simulink model "sampleModel366"  (R2021b)
settings: Solver=VariableStepAuto  StartTime=0.0  StopTime=10.0  RelTol=1e-3
undefined symbols (not defined in the file or in its folder): magnitude, Newton, Raphson
libraries: simulink x7, slpidlib x1
settings Model: Creator=user  LastModifiedBy=user

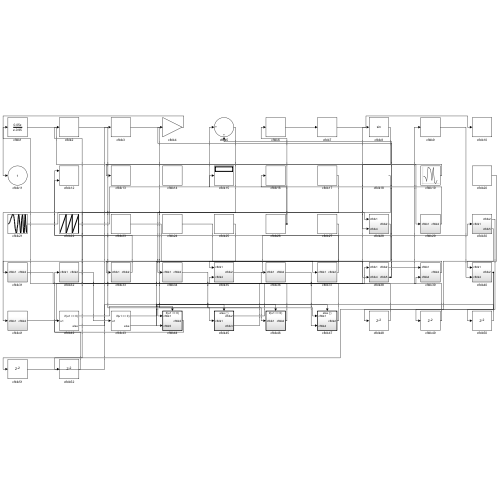
[thumbnail: Simulink's stored preview of the top-level diagram]
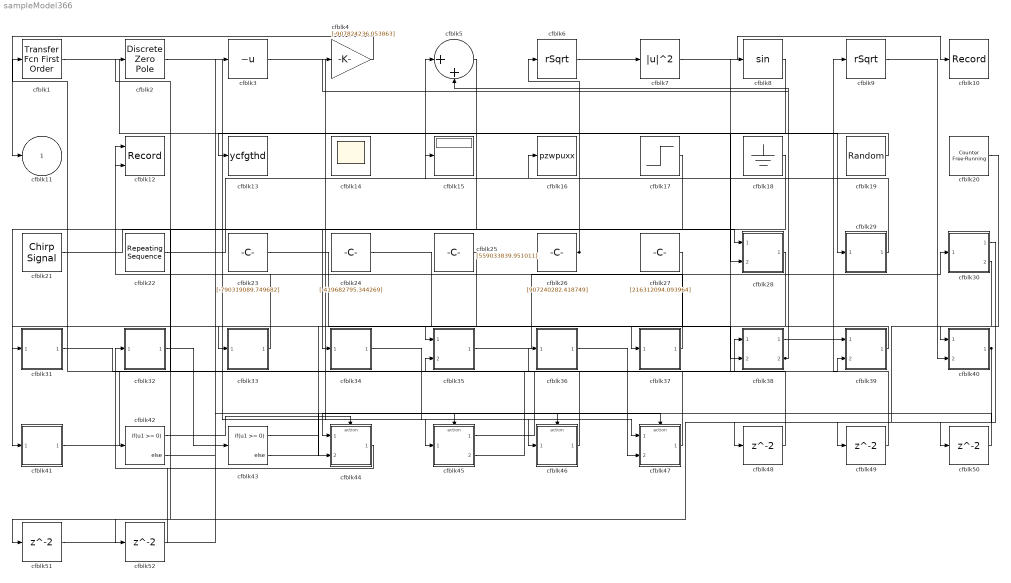
== system sampleModel366 ==
  cfblk1 : simulink/Discrete/Transfer Fcn First Order  PoleZ=0.95  ICPrevOutput=0.0  DoSatur=off
  cfblk10 : Record  FileSettingsInternal="{\"entries\":[{\"content\":{\"excelSettings\":{\"content\":{},\"type\":\"Streamout.ExcelSettings\"}},\"type\":\"Streamout.FileSettingStorage\",\"uuid\":\"b8f6fc41-c9ad-439a-b2d6-c8baa77482f0\"}],\"packageUris\":[\"http://schema.mathworks.com/mf0/streamout_blocks/R2020a\"],\"version\":\"1.0\"}"  SignalsInternal="{\"entries\":[{\"content\":{\"signals\":[{\"content\":{\"blockPath\":[\"sampleModel366/cfblk10\"],\"channel\":[],\"dimensions\":[1],\"domain\":\"sampleModel366/cfblk10\",\"lineColor\":\"#77ac30\",\"plots\":[1],\"port\":1,\"sid\":[\"\"],\"signalID\":15171,\"signalName\":\"cfblk7\"},\"type\":\"RecordBlkView.Signal\",\"uuid\":\"9359990c-ce8d-4281-8ced-0906e446bae2\"}]},\"type\":\"RecordBlkView.InputSignals\",\"uuid\":\"4aa2d466-194c-4383-9850-03db0f9c61d1\"}],\"packageUris\":[\"http://schema.mathworks.com/mf0/streamout_blocks/R2020a\"],\"version\":\"1.0\"}"  VisualizationBindings="{\"sparklinesplugin\":{\"info\":[{\"bindingParametersList\":[],\"subplotID\":1}]}}"
  cfblk12 : Record  FileSettingsInternal="{\"entries\":[{\"content\":{\"excelSettings\":{\"content\":{},\"type\":\"Streamout.ExcelSettings\"}},\"type\":\"Streamout.FileSettingStorage\",\"uuid\":\"68a24281-bd12-4afd-970e-6bf11612f610\"}],\"packageUris\":[\"http://schema.mathworks.com/mf0/streamout_blocks/R2020a\"],\"version\":\"1.0\"}"  Layout=[1 1]  SignalsInternal="{\"entries\":[{\"content\":{\"signals\":[{\"content\":{\"blockPath\":[\"sampleModel366/cfblk12\"],\"channel\":[],\"dimensions\":[1],\"domain\":\"sampleModel366/cfblk12\",\"lineColor\":\"#a2142f\",\"plots\":[1],\"port\":1,\"sid\":[\"\"],\"signalID\":15175,\"signalName\":\"cfblk37\"},\"type\":\"RecordBlkView.Signal\",\"uuid\":\"ee091272-d34b-41c7-8e6f-0fe17ae82c56\"},{\"content\":{\"blockPath\":[\"sampleModel366/cfblk12\"],\"channel\":[],\"dimensions\":[1],\"domain\":\"sampleModel366/cfblk12\",\"lineColor\":\"#139fff\",\"plots\":[1],\"port\":2,\"sid\":[\"\"],\"signalID\":15179,\"signalName\":\"cfblk33\"},\"type\":\"RecordBlkView.Signal\",\"uuid\":\"8b8a614a-960d-4b88-85a9-f6698a1653c2\"}]},\"type\":\"RecordBlkView.InputSignals\",\"uuid\":\"fcbbfd92-8274-4e20-9f39-c881c6846dea\"}],\"packageUris\":[\"http://schema.mathworks.com/mf0/streamout_blocks/R2020a\"],\"version\":\"1.0\"}"  VisualizationBindings="{\"xyplotplugin\":{\"info\":[{\"series\":[{\"bindingParametersList\":[{\"parameter\":\"X-Axis\",\"signalID\":15175,\"signalName\":\"cfblk37\"},{\"parameter\":\"Y-Axis\",\"signalID\":15179,\"signalName\":\"cfblk33\"}],\"seriesID\":23164}],\"subplotID\":1}]}}"  CompatibilityTag=XY
  cfblk13 : ToWorkspace  VariableName=ycfgthd  SaveFormat=Timeseries  SampleTime=-1
  cfblk14 : Scope
      settings: Floating=on
  cfblk15 : Display
  cfblk16 : ToWorkspace  VariableName=pzwpuxx  SaveFormat=Timeseries  SampleTime=-1
  cfblk17 : Step  Time=[5.000000]  Before=[178683344.473768]  After=[-623757983.996930]  SampleTime=0
  cfblk18 : Ground
  cfblk19 : RandomNumber  Mean=[-66694.921221]  Variance=[14545.838381]  Seed=[878185386.000000]  SampleTime=0.1
  cfblk2 : DiscreteZeroPole  Poles=[0 0.5]  Gain=1
  cfblk20 : simulink/Sources/Counter Free-Running  NumBits=[58.000000]  tsamp=-1
  cfblk21 : simulink/Sources/Chirp Signal  f1=[528864126.844984]  T=[-218465331.060448]  f2=[-783705554.218614]
  cfblk22 : simulink/Sources/Repeating Sequence  rep_seq_t=[0 2]  rep_seq_y=[169942996.806299, 363068189.269471]
  cfblk23 : Constant  Value=[-790319089.749682]  SampleTime=1
  cfblk24 : Constant  Value=[-419682795.344269]  SampleTime=1
  cfblk25 : Constant  Value=[559033839.951011]  SampleTime=1
  cfblk26 : Constant  Value=[907240282.418749]  SampleTime=1
  cfblk27 : Constant  Value=[216312094.093964]  SampleTime=1
  cfblk28 : Subsystem
  cfblk29 : Subsystem
  cfblk3 : UnaryMinus
  cfblk30 : Subsystem
  cfblk31 : Subsystem
  cfblk32 : Subsystem
  cfblk33 : Subsystem
  cfblk34 : Subsystem
  cfblk35 : Subsystem
  cfblk36 : Subsystem
  cfblk37 : Subsystem
  cfblk38 : Subsystem
  cfblk39 : Subsystem
  cfblk4 : Gain  Gain=[-907824236.053863]
  cfblk40 : Subsystem
  cfblk41 : Subsystem
  cfblk42 : If  IfExpression=u1 >= 0  SampleTime=1
  cfblk43 : If  IfExpression=u1 >= 0  SampleTime=1
  cfblk44 : Subsystem  TreatAsAtomicUnit=on
  cfblk45 : Subsystem  TreatAsAtomicUnit=on
  cfblk46 : Subsystem  TreatAsAtomicUnit=on
  cfblk47 : Subsystem  TreatAsAtomicUnit=on
  cfblk{48..52} (5 alike) : Delay  SampleTime=1
  cfblk5 : Sum  Inputs=|++
  cfblk6 : Sqrt  Operator=rSqrt  AlgorithmType=Newton-Raphson  SaturateOnIntegerOverflow=on
  cfblk7 : Math  Operator=magnitude^2  SaturateOnIntegerOverflow=on
  cfblk8 : Trigonometry
  cfblk9 : Sqrt  Operator=rSqrt  AlgorithmType=Newton-Raphson  SaturateOnIntegerOverflow=on
  cfblk11 : Outport
  wires:
  cfblk39/1(cfblk2) -> cfblk35/1(cfblk1)
  cfblk29/1(cfblk2) -> cfblk16/1
  cfblk2/1 -> cfblk47/1(cfblk1)
  cfblk7/1 -> cfblk10/1
  cfblk19/1 -> cfblk13/1
  cfblk44/1(cfblk2) -> cfblk32/1(cfblk1)
  cfblk6/1 -> cfblk7/1
  cfblk3/1 -> cfblk45/1(cfblk1)
  cfblk17/1 -> cfblk34/1(cfblk1)
  cfblk21/1 -> cfblk28/1(cfblk1)
  cfblk32/1(cfblk2) -> cfblk43/1
  cfblk22/1 -> cfblk5/1
  cfblk8/1 -> cfblk28/2(cfblk4)
  cfblk37/1(cfblk2) -> cfblk12/1
  cfblk1/1 -> cfblk29/1(cfblk1)
  cfblk36/1(cfblk2) -> cfblk47/2(cfblk4)
  cfblk4/1 -> cfblk11/1
  cfblk40/1(cfblk2) -> cfblk50/1, cfblk51/1
  cfblk24/1 -> cfblk37/1(cfblk1)
  cfblk18/1 -> cfblk41/1(cfblk1)
  cfblk46/1(cfblk2) -> cfblk2/1
  cfblk25/1 -> cfblk33/1(cfblk1)
  cfblk38/1(cfblk2) -> cfblk9/1
  cfblk27/1 -> cfblk44/2(cfblk5)
  cfblk20/1 -> cfblk40/1(cfblk1)
  cfblk26/1 -> cfblk15/1, cfblk6/1
  cfblk28/1(cfblk2) -> cfblk31/1(cfblk1)
  cfblk35/1(cfblk2) -> cfblk30/1(cfblk1)
  cfblk38/2(cfblk5) -> cfblk5/2, cfblk4/1
  cfblk47/1(cfblk2) -> cfblk1/1
  cfblk9/1 -> cfblk40/2(cfblk4)
  cfblk45/1(cfblk2) -> cfblk8/1
  cfblk33/1(cfblk2) -> cfblk12/2
  cfblk34/1(cfblk2) -> cfblk46/1(cfblk1)
  cfblk41/1(cfblk2) -> cfblk36/1(cfblk1)
  cfblk45/2(cfblk3) -> cfblk38/1(cfblk1)
  cfblk23/1 -> cfblk38/2(cfblk4)
  cfblk31/1(cfblk2) -> cfblk39/2(cfblk4)
  cfblk42/1 -> cfblk44/Action
  cfblk42/2 -> cfblk45/Action
  cfblk43/1 -> cfblk46/Action
  cfblk43/2 -> cfblk47/Action
  cfblk30/1(cfblk2) -> cfblk48/1
  cfblk48/1 -> cfblk35/2(cfblk4)
  cfblk30/2(cfblk5) -> cfblk49/1
  cfblk49/1 -> cfblk39/1(cfblk1)
  cfblk50/1 -> cfblk44/1(cfblk1)
  cfblk51/1 -> cfblk3/1
  cfblk5/1 -> cfblk52/1
  cfblk52/1 -> cfblk42/1

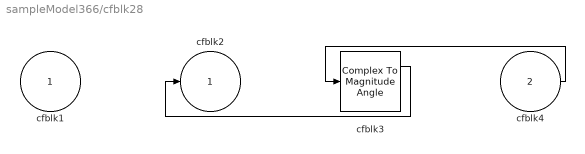
== system sampleModel366/cfblk28 ==
  cfblk1 : Inport
  cfblk4 : Inport  Port=2
  cfblk3 : ComplexToMagnitudeAngle
  cfblk2 : Outport
  wires:
  cfblk4/1 -> cfblk3/1
  cfblk3/1 -> cfblk2/1

== system sampleModel366/cfblk29 ==
  cfblk1 : Inport
  cfblk3 : simulink/Discrete/Transfer Fcn Lead or Lag  PoleZ=0.95  ZeroZ=0.75  ICPrevOutput=0.0  ICPrevInput=0.0  DoSatur=off
      settings: SourceProductBaseCode=SL
  cfblk2 : Outport
  wires:
  cfblk3/1 -> cfblk2/1
  cfblk1/1 -> cfblk3/1

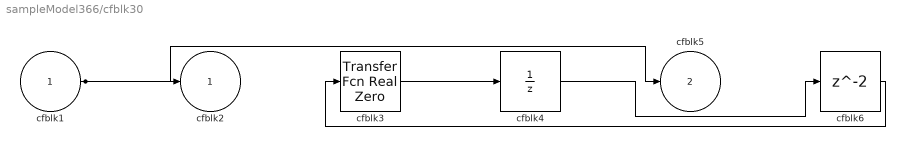
== system sampleModel366/cfblk30 ==
  cfblk1 : Inport
  cfblk3 : simulink/Discrete/Transfer Fcn Real Zero  ZeroZ=0.75  ICPrevInput=0.0  DoSatur=off
      settings: SourceProductBaseCode=SL
  cfblk4 : UnitDelay  HasFrameUpgradeWarning=on
  cfblk6 : Delay  SampleTime=1
  cfblk2 : Outport
  cfblk5 : Outport  Port=2
  wires:
  cfblk1/1 -> cfblk5/1, cfblk2/1
  cfblk3/1 -> cfblk4/1
  cfblk4/1 -> cfblk6/1
  cfblk6/1 -> cfblk3/1

== system sampleModel366/cfblk31 ==
  cfblk1 : Inport
  cfblk3 : Constant  Value=[900709185.564361]  SampleTime=1
  cfblk2 : Outport
  wires:
  cfblk1/1 -> cfblk2/1

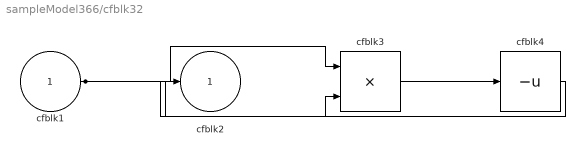
== system sampleModel366/cfblk32 ==
  cfblk1 : Inport
  cfblk3 : Product  Inputs=**
  cfblk4 : UnaryMinus
  cfblk2 : Outport
  wires:
  cfblk1/1 -> cfblk3/1, cfblk3/2
  cfblk4/1 -> cfblk2/1
  cfblk3/1 -> cfblk4/1

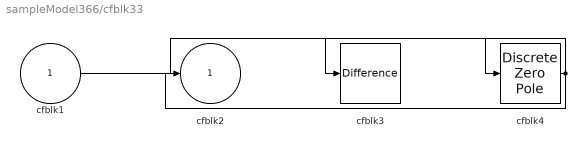
== system sampleModel366/cfblk33 ==
  cfblk1 : Inport
  cfblk3 : simulink/Discrete/Difference  ICPrevInput=0.0  OutMin=[]  OutMax=[]  OutDataTypeStr=Inherit: Inherit via back propagation  OutDataType=fixdt(1, 16)  OutScaling=2^-10  DoSatur=off
  cfblk4 : DiscreteZeroPole  Poles=[0 0.5]  Gain=1
  cfblk2 : Outport
  wires:
  cfblk1/1 -> cfblk4/1
  cfblk4/1 -> cfblk2/1, cfblk3/1

== system sampleModel366/cfblk34 ==
  cfblk1 : Inport
  cfblk3 : DiscreteTransferFcn  SampleTime=1
  cfblk2 : Outport
  wires:
  cfblk3/1 -> cfblk2/1
  cfblk1/1 -> cfblk3/1

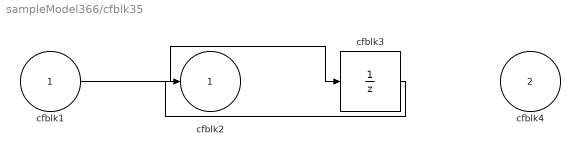
== system sampleModel366/cfblk35 ==
  cfblk1 : Inport
  cfblk4 : Inport  Port=2
  cfblk3 : UnitDelay  HasFrameUpgradeWarning=on
  cfblk2 : Outport
  wires:
  cfblk1/1 -> cfblk3/1
  cfblk3/1 -> cfblk2/1

== system sampleModel366/cfblk36 ==
  cfblk1 : Inport
  cfblk3 : Sum  Inputs=+-
  cfblk2 : Outport
  wires:
  cfblk1/1 -> cfblk3/1, cfblk3/2
  cfblk3/1 -> cfblk2/1

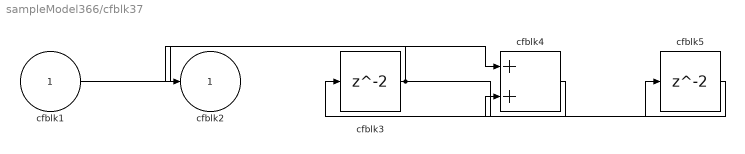
== system sampleModel366/cfblk37 ==
  cfblk1 : Inport
  cfblk3 : Delay  SampleTime=1
  cfblk4 : Sum
  cfblk5 : Delay  SampleTime=1
  cfblk2 : Outport
  wires:
  cfblk1/1 -> cfblk4/1
  cfblk3/1 -> cfblk2/1, cfblk5/1
  cfblk4/1 -> cfblk3/1
  cfblk5/1 -> cfblk4/2

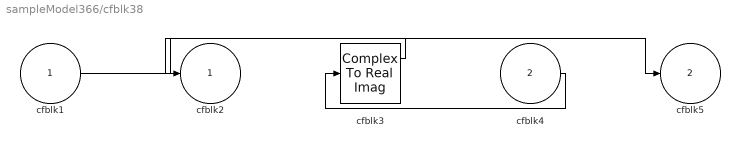
== system sampleModel366/cfblk38 ==
  cfblk1 : Inport
  cfblk4 : Inport  Port=2
  cfblk3 : ComplexToRealImag
  cfblk2 : Outport
  cfblk5 : Outport  Port=2
  wires:
  cfblk1/1 -> cfblk5/1
  cfblk4/1 -> cfblk3/1
  cfblk3/1 -> cfblk2/1

== system sampleModel366/cfblk39 ==
  cfblk1 : Inport
  cfblk4 : Inport  Port=2
  cfblk3 : Bias  Bias=[-463435880.451712]
  cfblk2 : Outport
  wires:
  cfblk1/1 -> cfblk2/1
  cfblk4/1 -> cfblk3/1

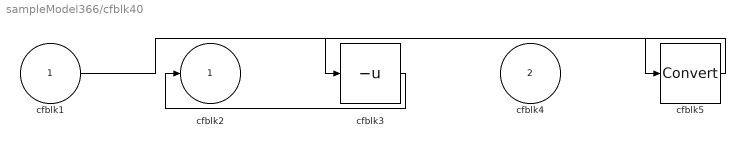
== system sampleModel366/cfblk40 ==
  cfblk1 : Inport
  cfblk4 : Inport  Port=2
  cfblk3 : UnaryMinus
  cfblk5 : DataTypeConversion
  cfblk2 : Outport
  wires:
  cfblk3/1 -> cfblk2/1
  cfblk1/1 -> cfblk5/1
  cfblk5/1 -> cfblk3/1

== system sampleModel366/cfblk41 ==
  cfblk1 : Inport
  cfblk3 : Sum  Inputs=--
  cfblk2 : Outport
  wires:
  cfblk1/1 -> cfblk3/1, cfblk3/2
  cfblk3/1 -> cfblk2/1

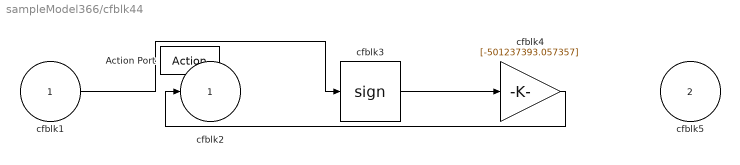
== system sampleModel366/cfblk44 ==
  cfblk1 : Inport
  cfblk5 : Inport  Port=2
  Action Port : ActionPort  ActionPortLabel=if(u1 >= 0)
  cfblk3 : Signum
  cfblk4 : Gain  Gain=[-501237393.057357]
  cfblk2 : Outport
  wires:
  cfblk4/1 -> cfblk2/1
  cfblk3/1 -> cfblk4/1
  cfblk1/1 -> cfblk3/1

== system sampleModel366/cfblk45 ==
  cfblk1 : Inport
  Action Port : ActionPort  ActionPortLabel=else
  cfblk2 : Outport
  cfblk3 : Outport  Port=2
  wires:
  cfblk1/1 -> cfblk3/1, cfblk2/1

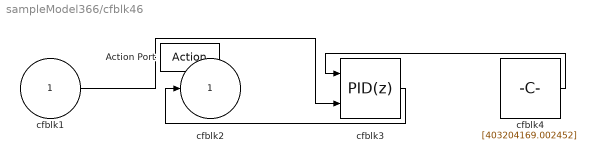
== system sampleModel366/cfblk46 ==
  cfblk1 : Inport
  Action Port : ActionPort  ActionPortLabel=if(u1 >= 0)
  cfblk3 : slpidlib/PID Controller (2DOF)  Controller=PID  Form=Parallel  TimeDomain=Discrete-time  UseExternalTs=off  SampleTime=-1  IntegratorMethod=Forward Euler  FilterMethod=Forward Euler  ControllerParametersSource=internal  P=1  I=1  D=0  UseFilter=on  N=100  b=1  c=1  TunerSelectOption=Transfer Function Based (PID Tuner App)  InitialConditionSource=internal  InitialConditionForIntegrator=0  InitialConditionForFilter=0  DifferentiatorICPrevScaledInput=0  ExternalReset=none  TrackingMode=off  Kt=1  LimitOutput=off  SatLimitsSource=internal  UpperSaturationLimit=inf  LowerSaturationLimit=-inf  LinearizeAsGain=off  AntiWindupMode=none  Kb=1  POutMin=[]  POutMax=[]  IOutMin=[]  IOutMax=[]  DOutMin=[]  DOutMax=[]  NOutMin=[]  NOutMax=[]  bOutMin=[]  bOutMax=[]  cOutMin=[]  cOutMax=[]  SumOutMin=[]  SumOutMax=[]  SaturationOutMin=[]  SaturationOutMax=[]  PParamMin=[]  PParamMax=[]  IParamMin=[]  IParamMax=[]  DParamMin=[]  DParamMax=[]  NParamMin=[]  NParamMax=[]  bParamMin=[]  bParamMax=[]  cParamMin=[]  cParamMax=[]  KbParamMin=[]  KbParamMax=[]  KtParamMin=[]  KtParamMax=[]  KbOutMin=[]  KbOutMax=[]  KtOutMin=[]  KtOutMax=[]  IntegratorOutMin=[]  IntegratorOutMax=[]  FilterOutMin=[]  FilterOutMax=[]  SumI1OutMin=[]  SumI1OutMax=[]  SumI2OutMin=[]  SumI2OutMax=[]  SumI3OutMin=[]  SumI3OutMax=[]  SumI4OutMin=[]  SumI4OutMax=[]  SumDOutMin=[]  SumDOutMax=[]  Sum1OutMin=[]  Sum1OutMax=[]  Sum2OutMin=[]  Sum2OutMax=[]  Sum3OutMin=[]  Sum3OutMax=[]  DifferentiatorOutMin=[]  DifferentiatorOutMax=[]  FilterDiffOutCoefMin=[]  FilterDiffOutCoefMax=[]  ReciprocalOutMin=[]  ReciprocalOutMax=[]  SumDenOutMin=[]  SumDenOutMax=[]  SumNumOutMin=[]  SumNumOutMax=[]  DivideOutMin=[]  DivideOutMax=[]  UdiffTsProdOutMin=[]  UdiffTsProdOutMax=[]  NTsProdOutMin=[]  NTsProdOutMax=[]  UintegralTsProdOutMin=[]  UintegralTsProdOutMax=[]  UngainTsProdOutMin=[]  UngainTsProdOutMax=[]  IntegratorContinuousStateAttributes=''  IntegratorStateMustResolveToSignalObject=off  IntegratorRTWStateStorageClass=Auto  FilterContinuousStateAttributes=''  FilterStateMustResolveToSignalObject=off  FilterRTWStateStorageClass=Auto  ParallelPVariant=InternalParameters  IdealPVariant=Disabled  IVariant=InternalParameters  DVariant=InternalParameters  bVariant=InternalParameters  cVariant=InternalParameters  IntegratorVariant=Discrete  SatVariant=Disabled  AWVariant=Passthrough  PCopyVariant=Disabled  TRVariant=Disabled  FdbkBlocksVariant=Forward  IdealPFdbkVariant=Disabled  SatFdbkVariant=Disabled  DerivativeFilterVariant=ForwardEulerFilter  NVariant=InternalParameters  NCopyVariant=Disabled  FilterICVariant=InternalICsFilter  IntegratorICVariant=InternalICs  ExternalResetVariant=Disabled  TRSumVariant=Passthrough  SumFdbkVariant=Disabled  SumVariant=Sum_PID  TsampFilterVariant=InternalTs  TsampNgainVariant=Passthrough  TsampIntegralVariant=Passthrough  ExternalSaturationOutDataTypeStr=Inherit: Same as second input
      settings: SourceProductBaseCode=SL
  cfblk4 : Constant  Value=[403204169.002452]  SampleTime=1
  cfblk2 : Outport
  wires:
  cfblk4/1 -> cfblk3/1
  cfblk3/1 -> cfblk2/1
  cfblk1/1 -> cfblk3/2

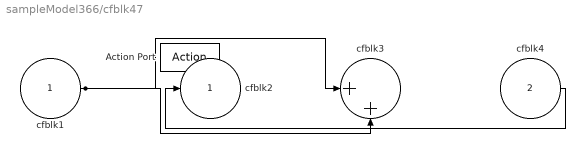
== system sampleModel366/cfblk47 ==
  cfblk1 : Inport
  cfblk4 : Inport  Port=2
  Action Port : ActionPort  ActionPortLabel=else
  cfblk3 : Sum  Inputs=|++
  cfblk2 : Outport
  wires:
  cfblk4/1 -> cfblk2/1
  cfblk1/1 -> cfblk3/1, cfblk3/2
